simulink model "wheelsdown_sim_pi_lead"  (R2018b)
settings: Solver=VariableStepAuto  StartTime=0.0  StopTime=5  RelTol=1e-3
values from neighbouring files (symbols this model uses):
  alpha = 0.20    (= 0.2)    [script.m]
  denum = [1 1904 6718]    [script.m]
  K_i = 1/tau_i    (= 714.285714286)    [script.m]
  K_p = 9.8855    [script.m]
  num = [6249]    [script.m]
  tau_d = 7.6316e-4    (= 0.00076316)    [script.m]
settings Model: Creator=megam  LastModifiedBy=megam

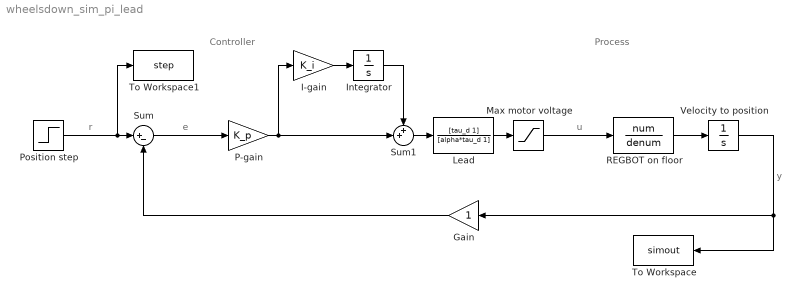
== system wheelsdown_sim_pi_lead ==
  note: r
  note: y
  note: u
  note: e
  note: Process
  note: Controller
  Gain : Gain
  I-gain : Gain  Gain=K_i
  Integrator : Integrator
  Lead : TransferFcn  Numerator=[tau_d 1]  Denominator=[alpha*tau_d 1]
  Max motor voltage : Saturate  UpperLimit=3  LowerLimit=-3
  P-gain : Gain  Gain=K_p
  Position step : Step  Time=0  After=0.5  SampleTime=0
  REGBOT on floor : TransferFcn  Numerator=num  Denominator=denum
  Sum : Sum  Inputs=|+-
  Sum1 : Sum  Inputs=++|
  To Workspace : ToWorkspace  VariableName=simout  SaveFormat=Timeseries  SampleTime=-1
  To Workspace1 : ToWorkspace  VariableName=step  SaveFormat=Timeseries  SampleTime=-1
  Velocity to position : Integrator
  wires:
  Position step/1 -> To Workspace1/1, Sum/1
  REGBOT on floor/1 -> Velocity to position/1
  Velocity to position/1 -> Gain/1, To Workspace/1
  Max motor voltage/1 -> REGBOT on floor/1
  I-gain/1 -> Integrator/1
  Integrator/1 -> Sum1/1
  Sum/1 -> P-gain/1
  P-gain/1 -> Sum1/2, I-gain/1
  Sum1/1 -> Lead/1
  Lead/1 -> Max motor voltage/1
  Gain/1 -> Sum/2
